simulink model "dspmidi"  (Simulink 8.3)
settings: Solver=FixedStepDiscrete  StartTime=0.0  StopTime=inf  FixedStep=1/44100  RelTol=1e-3
undefined symbols (not defined in the file or in its folder): Normalized
libraries: dspsrcs4 x11, dspmisc x1
Description:
  | Controlling Models Interactively with the MIDI Controls block
  | 
  | This demonstrates some simple ways the MIDI Controls block can be used
  | to interactively control Simulink(R) models
settings Model: Creator=The MathWorks Inc.
settings DataIOCC: LimitDataPoints=off  SaveOutput=off  SignalLogging=off  DSMLogging=off  SaveTime=off
settings OptimizationCC: ExpressionDepthLimit=2147483647
settings DebuggingCC: FcnCallInpInsideContextMsg=EnableAllAsWarning
settings GRTTargetCC: CombineOutputUpdateFcns=on  GRTInterface=off

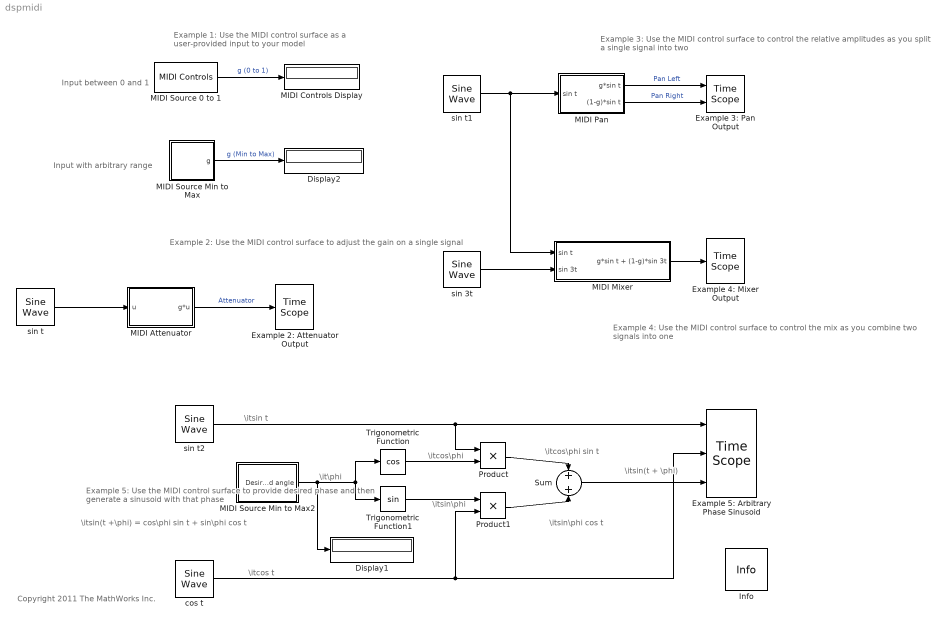
== system dspmidi ==
  note: \itsin(t +\phi) = cos\phi sin t + sin\phi cos t
  note: \itsin t
  note: \itcos t
  note: \itsin\phi cos t
  note: \itcos\phi sin t
  note: \itcos\phi
  note: \itsin\phi
  note: \itsin(t + \phi)
  note: \it\phi
  note: Example 1: Use the MIDI control surface
      | as a user-provided input to your model
  note: Input between 0 and 1
  note: Input with arbitrary range
  note: Example 2: Use the MIDI control surface to adjust the gain on a single signal
  note: Example 3: Use the MIDI control surface to control the relative
      | amplitudes as you split a single signal into two
  note: Example 4: Use the MIDI control surface to control the mix
      | as you combine two signals into one
  note: Example 5: Use the MIDI control surface to provide desired
      | phase and then generate a sinusoid with that phase
  note: Copyright 2011 The MathWorks Inc.
  Display1 : Display
  Display2 : Display
  Example 2: Attenuator Output : TimeScope  DefaultConfigurationName=spbscopes.TimeScopeBlockCfg  ScopeSpecification=DataTag0
  Example 3: Pan Output : TimeScope  NumInputPorts=2  DefaultConfigurationName=spbscopes.TimeScopeBlockCfg  ScopeSpecification=DataTag1
  Example 4: Mixer Output : TimeScope  DefaultConfigurationName=spbscopes.TimeScopeBlockCfg  ScopeSpecification=DataTag2
  Example 5: Arbitrary Phase Sinusoid : TimeScope  NumInputPorts=3  DefaultConfigurationName=spbscopes.TimeScopeBlockCfg  ScopeSpecification=DataTag3
  Info : dspmisc/Info  SystemSampleTime=-1
  MIDI Attenuator : Subsystem  mask{UseSpecifiedDevice=Default, DeviceName='', UseSpecifiedControls=Respond to any control, ControlNumbers=0, InitialValues=1, SyncAtStart=off}
      mask prompts: UseSpecifiedDevice "MIDI Device:"; DeviceName "MIDI device name:"; UseSpecifiedControls "MIDI controls:"; ControlNumbers "MIDI control numbers:"; InitialValues "Initial values:"; SyncAtStart "Send initial values to device at start"
      mask init:
      | set_param([gcb '/MIDI Controls'], 'UseSpecifiedDevice', get_param(gcb,'UseSpecifiedDevice'));
      | set_param([gcb '/MIDI Controls'], 'UseSpecifiedControls', get_param(gcb,'UseSpecifiedControls'));
      mask TypeOptions UseSpecifiedDevice: Default | Specify other
      mask Callback UseSpecifiedDevice:
      | switch 2*~isempty(strfind(get_param(gcbh,'UseSpecifiedDevice'),'pecif')) ...
      |         + ~isempty(strfind(get_param(gcbh,'UseSpecifiedControls'),'pecif'))
      |     case 0
      |         set_param(gcbh,'MaskVisibilities',{'on','off','on','off','on','on'});
      |     case 1
      |         set_param(gcbh,'MaskVisibilities',{'on','off','on','on','on','on'});
      |     case 2
      |         set_param(gcbh,'MaskVisibilities',{'on','on','on','off','on','on'});
      |     case 3
      |         set_param(gcbh,'MaskVisibilities',{'on','on','on','on','on','on'});
      | end
      mask TypeOptions DeviceName: MIDI Controls/DeviceName
      mask TypeOptions UseSpecifiedControls: Respond to any control | Respond to specified controls
      mask Callback UseSpecifiedControls:
      | switch 2*~isempty(strfind(get_param(gcbh,'UseSpecifiedDevice'),'pecif')) ...
      |         + ~isempty(strfind(get_param(gcbh,'UseSpecifiedControls'),'pecif'))
      |     case 0
      |         set_param(gcbh,'MaskVisibilities',{'on','off','on','off','on','on'});
      |     case 1
      |         set_param(gcbh,'MaskVisibilities',{'on','off','on','on','on','on'});
      |     case 2
      |         set_param(gcbh,'MaskVisibilities',{'on','on','on','off','on','on'});
      |     case 3
      |         set_param(gcbh,'MaskVisibilities',{'on','on','on','on','on','on'});
      | end
      mask TypeOptions ControlNumbers: MIDI Controls/ControlNumbers
      mask TypeOptions InitialValues: MIDI Controls/InitialValues
      mask TypeOptions SyncAtStart: MIDI Controls/SyncAtStart
  MIDI Controls Display : Display
  MIDI Mixer : Subsystem  mask{UseSpecifiedDevice=Default, DeviceName='', UseSpecifiedControls=Respond to any control, ControlNumbers=0, InitialValues=0.5, SyncAtStart=off}
      mask prompts: UseSpecifiedDevice "MIDI Device:"; DeviceName "MIDI device name:"; UseSpecifiedControls "MIDI controls:"; ControlNumbers "MIDI control numbers:"; InitialValues "Initial values:"; SyncAtStart "Send initial values to device at start"
      mask init:
      | set_param([gcb '/MIDI Controls'], 'UseSpecifiedDevice', get_param(gcb,'UseSpecifiedDevice'));
      | set_param([gcb '/MIDI Controls'], 'UseSpecifiedControls', get_param(gcb,'UseSpecifiedControls'));
      mask TypeOptions UseSpecifiedDevice: Default | Specify other
      mask Callback UseSpecifiedDevice:
      | switch 2*~isempty(strfind(get_param(gcbh,'UseSpecifiedDevice'),'pecif')) ...
      |         + ~isempty(strfind(get_param(gcbh,'UseSpecifiedControls'),'pecif'))
      |     case 0
      |         set_param(gcbh,'MaskVisibilities',{'on','off','on','off','on','on'});
      |     case 1
      |         set_param(gcbh,'MaskVisibilities',{'on','off','on','on','on','on'});
      |     case 2
      |         set_param(gcbh,'MaskVisibilities',{'on','on','on','off','on','on'});
      |     case 3
      |         set_param(gcbh,'MaskVisibilities',{'on','on','on','on','on','on'});
      | end
      mask TypeOptions DeviceName: MIDI Controls/DeviceName
      mask TypeOptions UseSpecifiedControls: Respond to any control | Respond to specified controls
      mask Callback UseSpecifiedControls:
      | switch 2*~isempty(strfind(get_param(gcbh,'UseSpecifiedDevice'),'pecif')) ...
      |         + ~isempty(strfind(get_param(gcbh,'UseSpecifiedControls'),'pecif'))
      |     case 0
      |         set_param(gcbh,'MaskVisibilities',{'on','off','on','off','on','on'});
      |     case 1
      |         set_param(gcbh,'MaskVisibilities',{'on','off','on','on','on','on'});
      |     case 2
      |         set_param(gcbh,'MaskVisibilities',{'on','on','on','off','on','on'});
      |     case 3
      |         set_param(gcbh,'MaskVisibilities',{'on','on','on','on','on','on'});
      | end
      mask TypeOptions ControlNumbers: MIDI Controls/ControlNumbers
      mask TypeOptions InitialValues: MIDI Controls/InitialValues
      mask TypeOptions SyncAtStart: MIDI Controls/SyncAtStart
  MIDI Pan : Subsystem  mask{UseSpecifiedDevice=Default, DeviceName='', UseSpecifiedControls=Respond to any control, ControlNumbers=0, InitialValues=0.5, SyncAtStart=off}
      mask prompts: UseSpecifiedDevice "MIDI Device:"; DeviceName "MIDI device name:"; UseSpecifiedControls "MIDI controls:"; ControlNumbers "MIDI control numbers:"; InitialValues "Initial values:"; SyncAtStart "Send initial values to device at start"
      mask init:
      | set_param([gcb '/MIDI Controls'], 'UseSpecifiedDevice', get_param(gcb,'UseSpecifiedDevice'));
      | set_param([gcb '/MIDI Controls'], 'UseSpecifiedControls', get_param(gcb,'UseSpecifiedControls'));
      mask TypeOptions UseSpecifiedDevice: Default | Specify other
      mask Callback UseSpecifiedDevice:
      | switch 2*~isempty(strfind(get_param(gcbh,'UseSpecifiedDevice'),'pecif')) ...
      |         + ~isempty(strfind(get_param(gcbh,'UseSpecifiedControls'),'pecif'))
      |     case 0
      |         set_param(gcbh,'MaskVisibilities',{'on','off','on','off','on','on'});
      |     case 1
      |         set_param(gcbh,'MaskVisibilities',{'on','off','on','on','on','on'});
      |     case 2
      |         set_param(gcbh,'MaskVisibilities',{'on','on','on','off','on','on'});
      |     case 3
      |         set_param(gcbh,'MaskVisibilities',{'on','on','on','on','on','on'});
      | end
      mask TypeOptions DeviceName: MIDI Controls/DeviceName
      mask TypeOptions UseSpecifiedControls: Respond to any control | Respond to specified controls
      mask Callback UseSpecifiedControls:
      | switch 2*~isempty(strfind(get_param(gcbh,'UseSpecifiedDevice'),'pecif')) ...
      |         + ~isempty(strfind(get_param(gcbh,'UseSpecifiedControls'),'pecif'))
      |     case 0
      |         set_param(gcbh,'MaskVisibilities',{'on','off','on','off','on','on'});
      |     case 1
      |         set_param(gcbh,'MaskVisibilities',{'on','off','on','on','on','on'});
      |     case 2
      |         set_param(gcbh,'MaskVisibilities',{'on','on','on','off','on','on'});
      |     case 3
      |         set_param(gcbh,'MaskVisibilities',{'on','on','on','on','on','on'});
      | end
      mask TypeOptions ControlNumbers: MIDI Controls/ControlNumbers
      mask TypeOptions InitialValues: MIDI Controls/InitialValues
      mask TypeOptions SyncAtStart: MIDI Controls/SyncAtStart
  MIDI Source 0 to 1 : dspsrcs4/MIDI Controls  UseSpecifiedDevice=Default  DeviceName=''  UseSpecifiedControls=Respond to any control  ControlNumbers=0  InitialValues=0  SyncAtStart=off  RawUint8=Normalized (0 - 1)
  MIDI Source Min to Max : Subsystem  mask{min=-pi, max=pi, UseSpecifiedDevice=Default, DeviceName='', UseSpecifiedControls=Respond to any control, ControlNumbers=0, InitialValues=0, SyncAtStart=off}
      mask prompts: UseSpecifiedDevice "MIDI Device:"; DeviceName "MIDI device name:"; UseSpecifiedControls "MIDI controls:"; ControlNumbers "MIDI control numbers:"; InitialValues "Initial values:"; SyncAtStart "Send initial values to device at start"
      mask init:
      | set_param([gcb '/MIDI Controls'], 'UseSpecifiedDevice', get_param(gcb,'UseSpecifiedDevice'));
      | set_param([gcb '/MIDI Controls'], 'UseSpecifiedControls', get_param(gcb,'UseSpecifiedControls'));
      mask TypeOptions UseSpecifiedDevice: Default	 | Specify other
      mask Callback UseSpecifiedDevice:
      | switch 2*~isempty(strfind(get_param(gcbh,'UseSpecifiedDevice'),'pecif')) ...
      |         + ~isempty(strfind(get_param(gcbh,'UseSpecifiedControls'),'pecif'))
      |     case 0
      |         set_param(gcbh,'MaskVisibilities',{'on','on','on','off','on','off','on','on'});
      |     case 1
      |         set_param(gcbh,'MaskVisibilities',{'on','on','on','off','on','on','on','on'});
      |     case 2
      |         set_param(gcbh,'MaskVisibilities',{'on','on','on','on','on','off','on','on'});
      |     case 3
      |         set_param(gcbh,'MaskVisibilities',{'on','on','on','on','on','on','on','on'});
      | end
      mask TypeOptions DeviceName: MIDI Controls/DeviceName
      mask TypeOptions UseSpecifiedControls: Respond to any control | Respond to specified controls
      mask Callback UseSpecifiedControls:
      | switch 2*~isempty(strfind(get_param(gcbh,'UseSpecifiedDevice'),'pecif')) ...
      |         + ~isempty(strfind(get_param(gcbh,'UseSpecifiedControls'),'pecif'))
      |     case 0
      |         set_param(gcbh,'MaskVisibilities',{'on','on','on','off','on','off','on','on'});
      |     case 1
      |         set_param(gcbh,'MaskVisibilities',{'on','on','on','off','on','on','on','on'});
      |     case 2
      |         set_param(gcbh,'MaskVisibilities',{'on','on','on','on','on','off','on','on'});
      |     case 3
      |         set_param(gcbh,'MaskVisibilities',{'on','on','on','on','on','on','on','on'});
      | end
      mask TypeOptions ControlNumbers: MIDI Controls/ControlNumbers
      mask TypeOptions SyncAtStart: MIDI Controls/SyncAtStart
  MIDI Source Min to Max2 : Subsystem  mask{min=-pi, max=pi, UseSpecifiedDevice=Default, DeviceName='', UseSpecifiedControls=Respond to any control, ControlNumbers=0, InitialValues=pi/4, SyncAtStart=off}
      mask prompts: UseSpecifiedDevice "MIDI Device:"; DeviceName "MIDI device name:"; UseSpecifiedControls "MIDI controls:"; ControlNumbers "MIDI control numbers:"; InitialValues "Initial values:"; SyncAtStart "Send initial values to device at start"
      mask init:
      | set_param([gcb '/MIDI Controls'], 'UseSpecifiedDevice', get_param(gcb,'UseSpecifiedDevice'));
      | set_param([gcb '/MIDI Controls'], 'UseSpecifiedControls', get_param(gcb,'UseSpecifiedControls'));
      mask TypeOptions UseSpecifiedDevice: Default	 | Specify other
      mask Callback UseSpecifiedDevice:
      | switch 2*~isempty(strfind(get_param(gcbh,'UseSpecifiedDevice'),'pecif')) ...
      |         + ~isempty(strfind(get_param(gcbh,'UseSpecifiedControls'),'pecif'))
      |     case 0
      |         set_param(gcbh,'MaskVisibilities',{'on','on','on','off','on','off','on','on'});
      |     case 1
      |         set_param(gcbh,'MaskVisibilities',{'on','on','on','off','on','on','on','on'});
      |     case 2
      |         set_param(gcbh,'MaskVisibilities',{'on','on','on','on','on','off','on','on'});
      |     case 3
      |         set_param(gcbh,'MaskVisibilities',{'on','on','on','on','on','on','on','on'});
      | end
      mask TypeOptions DeviceName: MIDI Controls/DeviceName
      mask TypeOptions UseSpecifiedControls: Respond to any control | Respond to specified controls
      mask Callback UseSpecifiedControls:
      | switch 2*~isempty(strfind(get_param(gcbh,'UseSpecifiedDevice'),'pecif')) ...
      |         + ~isempty(strfind(get_param(gcbh,'UseSpecifiedControls'),'pecif'))
      |     case 0
      |         set_param(gcbh,'MaskVisibilities',{'on','on','on','off','on','off','on','on'});
      |     case 1
      |         set_param(gcbh,'MaskVisibilities',{'on','on','on','off','on','on','on','on'});
      |     case 2
      |         set_param(gcbh,'MaskVisibilities',{'on','on','on','on','on','off','on','on'});
      |     case 3
      |         set_param(gcbh,'MaskVisibilities',{'on','on','on','on','on','on','on','on'});
      | end
      mask TypeOptions ControlNumbers: MIDI Controls/ControlNumbers
      mask TypeOptions SyncAtStart: MIDI Controls/SyncAtStart
  Product : Product  RndMeth=Zero
  Product1 : Product  RndMeth=Zero
  Sum : Sum
  Trigonometric Function : Trigonometry  Operator=cos
  Trigonometric Function1 : Trigonometry
  cos t : dspsrcs4/Sine Wave  Amplitude=1  Frequency=44100/256  Phase=pi/2  SampleMode=Discrete  OutComplex=Real  CompMethod=Trigonometric fcn  TableSize=Speed  SampleTime=1/44100  SamplesPerFrame=256  ResetState=Restart at time zero  dataType=double  wordLen=16  udDataType=sfix(16)  fracBitsMode=Best precision  numFracBits=15  OutDataTypeStr=double  LastOutDataTypeStr=double
  sin 3t : dspsrcs4/Sine Wave  Amplitude=1  Frequency=3*44100/(256)  Phase=0  SampleMode=Discrete  OutComplex=Real  CompMethod=Trigonometric fcn  TableSize=Speed  SampleTime=1/44100  SamplesPerFrame=256  ResetState=Restart at time zero  dataType=double  wordLen=16  udDataType=sfix(16)  fracBitsMode=Best precision  numFracBits=15  OutDataTypeStr=double  LastOutDataTypeStr=double
  sin t : dspsrcs4/Sine Wave  Amplitude=1  Frequency=44100/256  Phase=0  SampleMode=Discrete  OutComplex=Real  CompMethod=Trigonometric fcn  TableSize=Speed  SampleTime=1/44100  SamplesPerFrame=256  ResetState=Restart at time zero  dataType=double  wordLen=16  udDataType=sfix(16)  fracBitsMode=Best precision  numFracBits=15  OutDataTypeStr=double  LastOutDataTypeStr=double
  sin t1 : dspsrcs4/Sine Wave  Amplitude=1  Frequency=44100/256  Phase=0  SampleMode=Discrete  OutComplex=Real  CompMethod=Trigonometric fcn  TableSize=Speed  SampleTime=1/44100  SamplesPerFrame=256  ResetState=Restart at time zero  dataType=double  wordLen=16  udDataType=sfix(16)  fracBitsMode=Best precision  numFracBits=15  OutDataTypeStr=double  LastOutDataTypeStr=double
  sin t2 : dspsrcs4/Sine Wave  Amplitude=1  Frequency=44100/256  Phase=0  SampleMode=Discrete  OutComplex=Real  CompMethod=Trigonometric fcn  TableSize=Speed  SampleTime=1/44100  SamplesPerFrame=256  ResetState=Restart at time zero  dataType=double  wordLen=16  udDataType=sfix(16)  fracBitsMode=Best precision  numFracBits=15  OutDataTypeStr=double  LastOutDataTypeStr=double
  wires:
  Trigonometric Function1/1 -> Product1/1
  Trigonometric Function/1 -> Product/2
  Product/1 -> Sum/1
  cos t/1 -> Product1/2, Example 5: Arbitrary Phase Sinusoid/2
  Product1/1 -> Sum/2
  MIDI Source Min to Max2/1(Desired angle) -> Trigonometric Function1/1, Trigonometric Function/1, Display1/1
  MIDI Source 0 to 1/1 -> MIDI Controls Display/1  "g (0 to 1)"
  Sum/1 -> Example 5: Arbitrary Phase Sinusoid/3
  sin t2/1 -> Product/1, Example 5: Arbitrary Phase Sinusoid/1
  MIDI Source Min to Max/1(g) -> Display2/1  "g (Min to Max)"
  sin t/1 -> MIDI Attenuator/1(u)
  MIDI Attenuator/1(g*u) -> Example 2: Attenuator Output/1  "Attenuator"
  MIDI Pan/1(g*sin t) -> Example 3: Pan Output/1  "Pan Left"
  MIDI Pan/2((1-g)*sin t) -> Example 3: Pan Output/2  "Pan Right"
  sin 3t/1 -> MIDI Mixer/2(sin 3t)
  MIDI Mixer/1(g*sin t + (1-g)*sin 3t) -> Example 4: Mixer Output/1
  sin t1/1 -> MIDI Pan/1(sin t), MIDI Mixer/1(sin t)

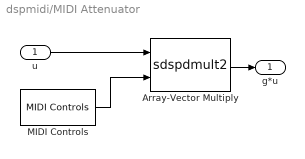
== system dspmidi/MIDI Attenuator ==
  u : Inport
  Array-Vector Multiply : S-Function  DialogController=dspDDGCreate  DialogControllerArgs=DataTag4  FunctionName=sdspdmult2  Parameters=1,Dimension,V_Source,V_VectFromMask,firstCoeffMin,firstCoeffMax,outputMin,outputMax,dtInfo.firstCoeffMode,dtInfo.firstCoeffWordLength,dtInfo.firstCoeffFracLength,dtInfo.prodOutputMode,dtInfo.prodOutputWordLength,dtInfo.prodOutputFracLength,dtInfo.accumMode,dtInfo.accumWordLength,dtInfo.accumFracLength,dtInfo.outputMode,dtInfo.outputWordLength,dtInfo.outputFracLength,dtInfo.roundingMode,dtInfo.overflowMode  EnableBusSupport=off  mask(Array-Vector Multiply){mode=Mute, saveAsFlag=0, Dimension=2, V_Source=Input port, V_VectFromMask=[0.5 0.25], additionalParams=off, allowOverrides=on, firstCoeffMode=Same word length as input, firstCoeffSignedness=Auto, firstCoeffWordLength=16, firstCoeffFracLength=15, firstCoeffDataTypeStr=Inherit: Same word length as input, firstCoeffLastDataTypeStr=Inherit: Same word length as input, firstCoeffMin=[], firstCoeffMax=[], outputMode=Same as product output, outputSignedness=Auto, outputWordLength=16, outputFracLength=15, outputDataTypeStr=Inherit: Same as product output, outputLastDataTypeStr=Inherit: Same as product output, outputMin=[], outputMax=[], accumMode=Inherit via internal rule, accumSignedness=Auto, accumWordLength=32, accumFracLength=30, accumDataTypeStr=Inherit: Inherit via internal rule, accumLastDataTypeStr=Inherit: Inherit via internal rule, prodOutputMode=Inherit via internal rule, prodOutputSignedness=Auto, prodOutputWordLength=32, prodOutputFracLength=30, prodOutputDataTypeStr=Inherit: Inherit via internal rule, prodOutputLastDataTypeStr=Inherit: Inherit via internal rule, roundingMode=Floor, overflowMode=off, LockScale=off}
      mask prompts: saveAsFlag "Save_as flag:"; Dimension "Multiply along dimension:"; V_Source "Vector (V) source:"; V_VectFromMask "Vector (V):"; additionalParams "------- Show additional parameters -------"; allowOverrides "Allow overrides from DSP Fixed-Point Attributes blocks"; firstCoeffMode "Fixed-point scaling vector attributes:"; firstCoeffSignedness "Scaling vector elements signedness:"; firstCoeffWordLength "Scaling vector elements word length:"; firstCoeffFracLength "Scaling vector elements fraction length:"; firstCoeffDataTypeStr "Vector (V) data type string:"; firstCoeffLastDataTypeStr "Last vector (V) data type string:"; firstCoeffMin "Last vector (V) minimum:"; firstCoeffMax "Last vector (V) maximum:"; outputMode "Fixed-point output attributes:"; outputSignedness "Output signedness:"; outputWordLength "Output word length:"; outputFracLength "Output fraction length:"; outputDataTypeStr "Output data type string:"; outputLastDataTypeStr "Last output data type string:"; outputMin "Output minimum:"; outputMax "Output maximum:"; accumMode "Fixed-point accumulator attributes:"; accumSignedness "Accumulator signedness:"; accumWordLength "Accumulator word length"; accumFracLength "Accumulator fraction length:"; accumDataTypeStr "Accum data type string:"; accumLastDataTypeStr "Last accum data type string:"; prodOutputMode "Fixed-point product output attributes:"; prodOutputSignedness "Product output signedness:"; prodOutputWordLength "Product output word length:"; prodOutputFracLength "Product output fraction length:"; prodOutputDataTypeStr "ProdOutput data type string:"; prodOutputLastDataTypeStr "Last prodOutput data type string:"; roundingMode "Round integer calculations toward:"; overflowMode "Saturate on integer overflow"; LockScale "Lock scaling"
      mask help: Multiply the input array A by the elements of vector V along the specified dimension. In the two-dimensional case, this is equivalent to multiplying a full matrix (A) by a diagonal (V). Note that unoriented input signals are treated as oriented column vectors. The output of this block is always oriented.
      mask init:
      | blkh = gcbh;
      | m    = get_param(blkh, 'mode');
      | if (~strcmp(m, 'Mute'))
      |     if (saveAsFlag == 0)
      |         if strcmp(m,'Scale rows (D*A)')
      |             set_param(blkh, 'Dimension', '1', 'mode', 'Mute');
      |         elseif strcmp(m,'Scale columns (A*D)')
      |             set_param(blkh, 'Dimension', '2', 'mode', 'Mute');
      |         end
      |     end
      | end
      | dtRows = dspblkGetArrayVectorMpyDTRowInfo();
      | dtInfo = dspGetUDTFixptDataTypeInfo(blkh, dtRows, true);
      mask Help: eval('blocksethelp');
      mask TypeOptions mode: Scale rows (D*A) | Scale columns (A*D) | Mute
      mask TypeOptions V_Source: Input port | Dialog parameter
      mask TypeOptions firstCoeffMode: Same word length as input | Specify word length | Binary point scaling | Slope and bias scaling | User-defined
      mask TypeOptions firstCoeffSignedness: Auto | Signed
      mask TypeOptions outputMode: Same as product output | Same as first input | Binary point scaling | Slope and bias scaling | User-defined
      mask TypeOptions outputSignedness: Auto | Signed
      mask TypeOptions accumMode: Inherit via internal rule | Same as product output | Same as first input | Binary point scaling | Slope and bias scaling | User-defined
      mask TypeOptions accumSignedness: Auto | Signed
      mask TypeOptions prodOutputMode: Inherit via internal rule | Same as first input | Binary point scaling | Slope and bias scaling | User-defined
      mask TypeOptions prodOutputSignedness: Auto | Signed
      mask TypeOptions roundingMode: Ceiling | Convergent | Floor | Nearest | Round | Simplest | Zero
      mask Display:
      | inp1_index = 1;
      | inp1_label = 'A';
      | if (V_Source == 1),
      |   inp2_index = 2;
      |   inp2_label = 'V';
      | else
      |   inp2_index = 1;
      |   inp2_label = 'A';
      | end
      | 
      | port_label('input',inp1_index,inp1_label);
      | port_label('input',inp2_index,inp2_label);
      | disp('Array-Vector\nMultiply');
  MIDI Controls : dspsrcs4/MIDI Controls  UseSpecifiedDevice=Default  DeviceName=DeviceName  UseSpecifiedControls=Respond to any control  ControlNumbers=ControlNumbers  InitialValues=InitialValues  SyncAtStart=off  RawUint8=Normalized (0 - 1)
  g*u : Outport
  wires:
  Array-Vector Multiply/1 -> g*u/1
  u/1 -> Array-Vector Multiply/1
  MIDI Controls/1 -> Array-Vector Multiply/2

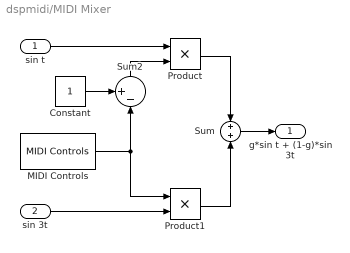
== system dspmidi/MIDI Mixer ==
  sin t : Inport
  sin 3t : Inport  Port=2
  Constant : Constant
  MIDI Controls : dspsrcs4/MIDI Controls  UseSpecifiedDevice=Default  DeviceName=DeviceName  UseSpecifiedControls=Respond to any control  ControlNumbers=ControlNumbers  InitialValues=InitialValues  SyncAtStart=off  RawUint8=Normalized (0 - 1)
  Product : Product  RndMeth=Zero
  Product1 : Product  RndMeth=Zero
  Sum : Sum
  Sum2 : Sum  Inputs=+-|
  g*sin t + (1-g)*sin 3t : Outport
  wires:
  Sum2/1 -> Product/2
  Constant/1 -> Sum2/1
  Product1/1 -> Sum/2
  sin 3t/1 -> Product1/2
  Product/1 -> Sum/1
  Sum/1 -> g*sin t + (1-g)*sin 3t/1
  MIDI Controls/1 -> Product1/1, Sum2/2
  sin t/1 -> Product/1

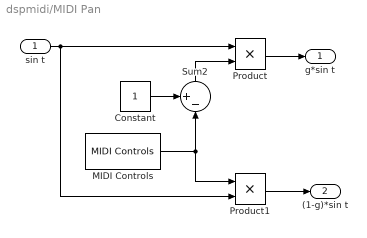
== system dspmidi/MIDI Pan ==
  sin t : Inport
  Constant : Constant
  MIDI Controls : dspsrcs4/MIDI Controls  UseSpecifiedDevice=Default  DeviceName=DeviceName  UseSpecifiedControls=Respond to any control  ControlNumbers=ControlNumbers  InitialValues=InitialValues  SyncAtStart=off  RawUint8=Normalized (0 - 1)
  Product : Product  RndMeth=Zero
  Product1 : Product  RndMeth=Zero
  Sum2 : Sum  Inputs=+-|
  g*sin t : Outport
  (1-g)*sin t : Outport  Port=2
  wires:
  Sum2/1 -> Product/2
  Constant/1 -> Sum2/1
  MIDI Controls/1 -> Product1/1, Sum2/2
  sin t/1 -> Product/1, Product1/2
  Product/1 -> g*sin t/1
  Product1/1 -> (1-g)*sin t/1

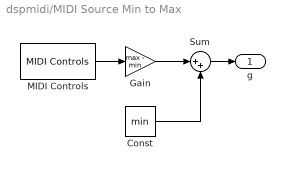
== system dspmidi/MIDI Source Min to Max ==
  Const : Constant  Value=min
  Gain : Gain  Gain=max - min
  MIDI Controls : dspsrcs4/MIDI Controls  UseSpecifiedDevice=Default  DeviceName=DeviceName  UseSpecifiedControls=Respond to any control  ControlNumbers=ControlNumbers  InitialValues=(InitialValues-min)./(max-min)  SyncAtStart=off  RawUint8=Normalized (0 - 1)
  Sum : Sum  Inputs=|++
  g : Outport
  wires:
  Sum/1 -> g/1
  MIDI Controls/1 -> Gain/1
  Const/1 -> Sum/2
  Gain/1 -> Sum/1

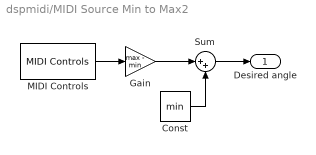
== system dspmidi/MIDI Source Min to Max2 ==
  Const : Constant  Value=min
  Gain : Gain  Gain=max - min
  MIDI Controls : dspsrcs4/MIDI Controls  UseSpecifiedDevice=Default  DeviceName=DeviceName  UseSpecifiedControls=Respond to any control  ControlNumbers=ControlNumbers  InitialValues=(InitialValues-min)./(max-min)  SyncAtStart=off  RawUint8=Normalized (0 - 1)
  Sum : Sum  Inputs=|++
  Desired angle : Outport
  wires:
  Gain/1 -> Sum/1
  Const/1 -> Sum/2
  MIDI Controls/1 -> Gain/1
  Sum/1 -> Desired angle/1
